simulink model "dampingfactor"  (R2026a)
settings: Solver=VariableStepAuto
settings Model: Creator=tanmay  LastModifiedBy=tanmay

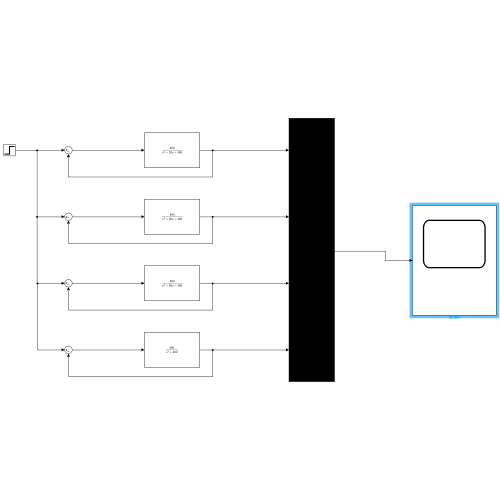
[thumbnail: Simulink's stored preview of the top-level diagram]
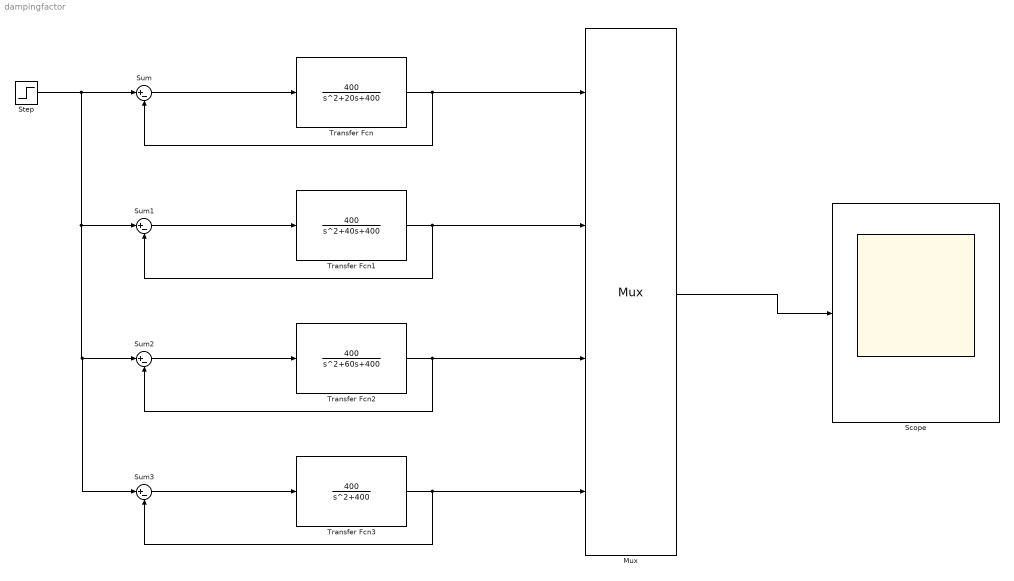
== system dampingfactor ==
  Mux : Mux
  Scope : Scope
      settings: ActiveDisplayYMinimum=-0.12485567034662236  ActiveDisplayYMaximum=1.1237010331196016
  Step : Step  SampleTime=0
  Sum{,1..3} (4 alike) : Sum  Inputs=|+-
  Transfer Fcn : TransferFcn  Numerator=[400]  Denominator=[1 20 400]
  Transfer Fcn1 : TransferFcn  Numerator=[400]  Denominator=[1 40 400]
  Transfer Fcn2 : TransferFcn  Numerator=[400]  Denominator=[1 60 400]
  Transfer Fcn3 : TransferFcn  Numerator=[400]  Denominator=[1 0 400]
  wires:
  Mux/1 -> Scope/1
  Transfer Fcn/1 -> Sum/2, Mux/1
  Sum/1 -> Transfer Fcn/1
  Step/1 -> Sum3/1, Sum2/1, Sum1/1, Sum/1
  Transfer Fcn1/1 -> Mux/2, Sum1/2
  Sum1/1 -> Transfer Fcn1/1
  Transfer Fcn2/1 -> Mux/3, Sum2/2
  Sum2/1 -> Transfer Fcn2/1
  Transfer Fcn3/1 -> Mux/4, Sum3/2
  Sum3/1 -> Transfer Fcn3/1
